simulink model "Progetto_Tesi"  (R2023b)
settings: Solver=VariableStepAuto  StartTime=0.0  StopTime=inf  RelTol=1e-3
StartFcn:
  | model_params
model workspace (MAT data in the model file):
  ax_pre_init = 7
values from neighbouring files (symbols this model uses):
  soglia_nonlin = 0.5    [model_params.m]
undefined symbols (not defined in the file or in its folder): deg, m, s
libraries: qbmove_library x4, CP_library x1, QB_pacer_lib x1
settings Model: Creator=ilari  LastModifiedBy=ilari

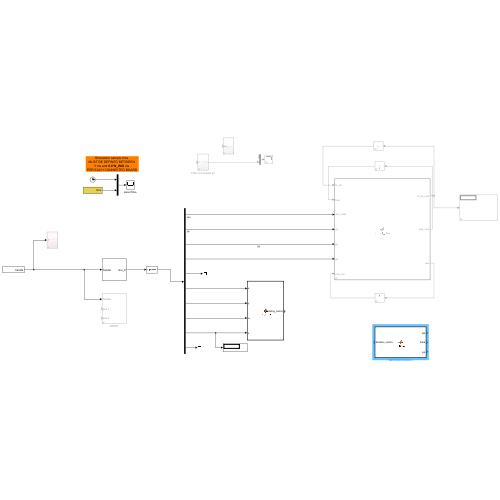
[thumbnail: Simulink's stored preview of the top-level diagram]
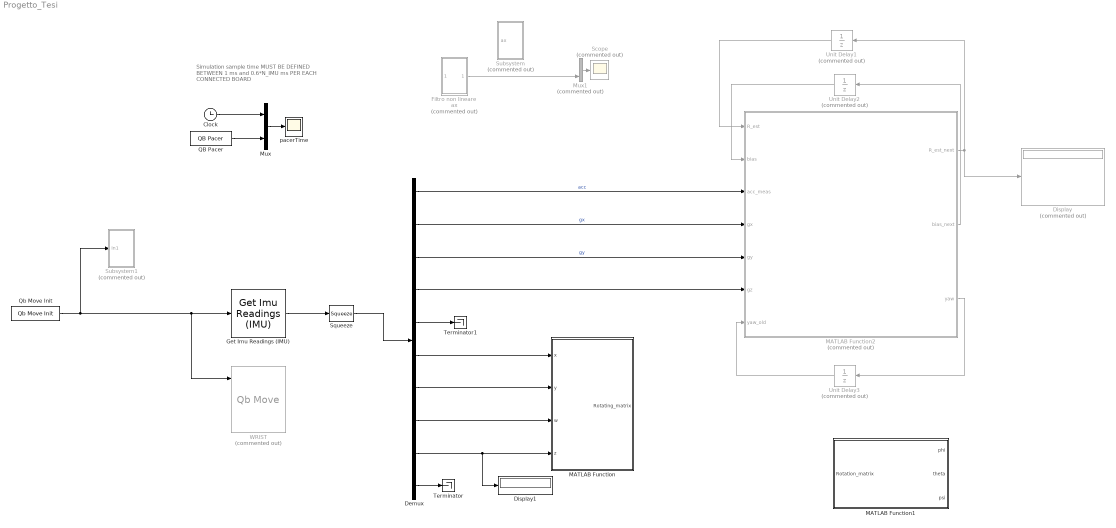
== system Progetto_Tesi ==
  note: Simulation sample time
      | MUST BE DEFINED BETWEEN
      | 1 ms and 0.6*N_IMU ms
      | PER EACH CONNECTED BOARD
  Clock : Clock
  Demux : Demux  Outputs=[3 1 1 1 3 1 1 1 1 1]
  Display : Display  Commented=on
  Display1 : Display
  Filtro non lineare ax : Subsystem  Commented=on
  Get Imu Readings (IMU) : CP_library/Get Imu Readings (IMU)  ID=2  N_IMU=1  DAISY_CHAINING=off  ACC_UNITY=m/(s^2)  GYRO_UNITY=deg/s  MAG_UNITY=uT
      settings: SourceProductName=Centro Piaggio Library
  MATLAB Function : MATLAB Function  TreatAsAtomicUnit=on
  MATLAB Function1 : MATLAB Function  TreatAsAtomicUnit=on
  MATLAB Function2 : MATLAB Function  Commented=on  TreatAsAtomicUnit=on
  Mux : Mux  Inputs=2
  Mux1 : Mux  Commented=on  Inputs=2
  QB Pacer : QB_pacer_lib/QB Pacer  simTimePerRealTime=1
      settings: SourceProductName=QB Pacer
  Qb Move Init : qbmove_library/Qb Move Init  NUMBER_OF_COM='COM9'  BAUD_RATE_COM=2000000
      settings: SourceProductName=Qb Move Library
  Scope : Scope  Commented=on
  Squeeze : Squeeze
  Subsystem : Subsystem  Commented=on
  Subsystem1 : Subsystem  Commented=on
  Terminator : Terminator
  Terminator1 : Terminator
  Unit Delay1 : UnitDelay  Commented=on  SampleTime=-1  HasFrameUpgradeWarning=on
  Unit Delay2 : UnitDelay  Commented=on  SampleTime=-1  HasFrameUpgradeWarning=on
  Unit Delay3 : UnitDelay  Commented=on  SampleTime=-1  HasFrameUpgradeWarning=on
  WRIST : qbmove_library/Qb Move  Commented=on  ID=2  ACTIVE_COMM_DIRECTIONS=Tx  CONTROL_MODE=Prime Movers Positions  DAISY_CHAINING=off  MAX_ANG=0  SW_LIMIT=inf  OFFSET=0  ACTIVATE=on  WDT=0.0  UNIT=TICK
      settings: SourceProductName=Qb Move Library
  pacerTime : Scope
  wires:
  Clock/1 -> Mux/1
  QB Pacer/1 -> Mux/2
  Mux/1 -> pacerTime/1
  Qb Move Init/1 -> Get Imu Readings (IMU)/1, WRIST/1, Subsystem1/1(In1)
  Get Imu Readings (IMU)/1 -> Squeeze/1
  Squeeze/1 -> Demux/1
  Filtro non lineare ax/1(Out1) -> Mux1/2
  Mux1/1 -> Scope/1
  Demux/1 -> MATLAB Function2/3(acc_meas)  "acc"
  Demux/2 -> MATLAB Function2/4(gx)  "gx"
  Demux/3 -> MATLAB Function2/5(gy)  "gy"
  Demux/4 -> MATLAB Function2/6(gz)
  MATLAB Function2/3(yaw) -> Unit Delay3/1
  Unit Delay3/1 -> MATLAB Function2/7(yaw_old)
  MATLAB Function2/2(bias_next) -> Unit Delay2/1
  Unit Delay2/1 -> MATLAB Function2/2(bias)
  Unit Delay1/1 -> MATLAB Function2/1(R_est)
  MATLAB Function2/1(R_est_next) -> Unit Delay1/1, Display/1
  Demux/5 -> Terminator1/1
  Demux/10 -> Terminator/1
  Demux/6 -> MATLAB Function/1(x)
  Demux/7 -> MATLAB Function/2(y)
  Demux/8 -> MATLAB Function/3(w)
  Demux/9 -> Display1/1, MATLAB Function/4(z)

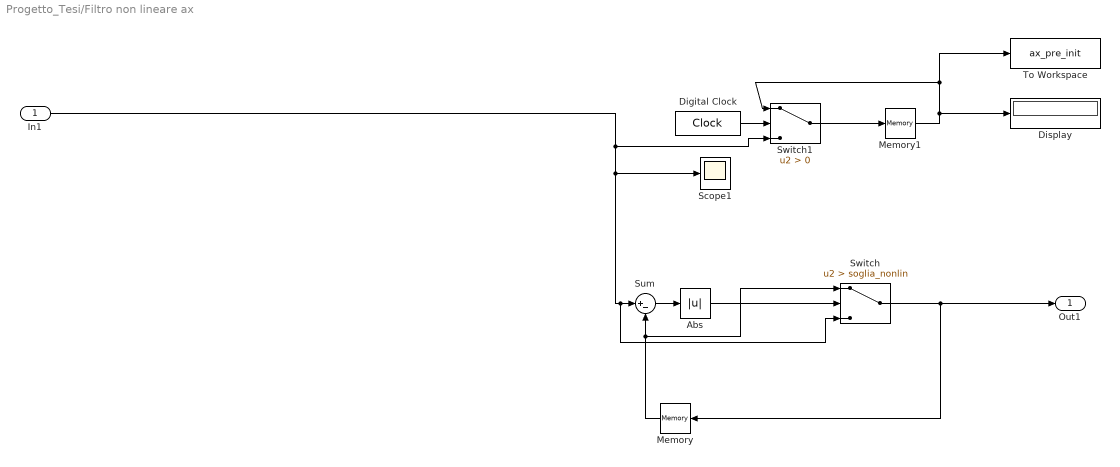
== system Progetto_Tesi/Filtro non lineare ax ==
  In1 : Inport
  Abs : Abs  SaturateOnIntegerOverflow=off
  Digital Clock : DigitalClock
  Display : Display
  Memory : Memory  InitialCondition=ax_pre_init
  Memory1 : Memory
  Scope1 : Scope
  Sum : Sum  Inputs=|+-
  Switch : Switch  Criteria=u2 > Threshold  Threshold=soglia_nonlin  SaturateOnIntegerOverflow=off  InputSameDT=off
  Switch1 : Switch  Criteria=u2 > Threshold  SaturateOnIntegerOverflow=off  InputSameDT=off
  To Workspace : ToWorkspace  VariableName=ax_pre_init  SaveFormat=Timeseries  SampleTime=-1
  Out1 : Outport
  wires:
  Switch/1 -> Out1/1, Memory/1
  Memory/1 -> Sum/2, Switch/1
  In1/1 -> Switch1/3, Switch/3, Sum/1, Scope1/1
  Abs/1 -> Switch/2
  Sum/1 -> Abs/1
  Switch1/1 -> Memory1/1
  Memory1/1 -> Switch1/1, To Workspace/1, Display/1
  Digital Clock/1 -> Switch1/2

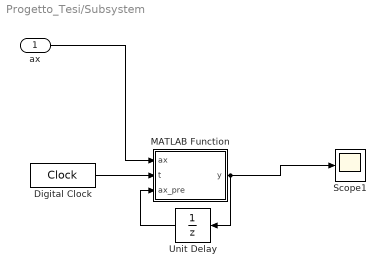
== system Progetto_Tesi/Subsystem ==
  ax : Inport
  Digital Clock : DigitalClock
  MATLAB Function : MATLAB Function  TreatAsAtomicUnit=on
  Scope1 : Scope
  Unit Delay : UnitDelay  SampleTime=-1  HasFrameUpgradeWarning=on
  wires:
  MATLAB Function/1(y) -> Unit Delay/1, Scope1/1
  Digital Clock/1 -> MATLAB Function/2(t)
  Unit Delay/1 -> MATLAB Function/3(ax_pre)
  ax/1 -> MATLAB Function/1(ax)

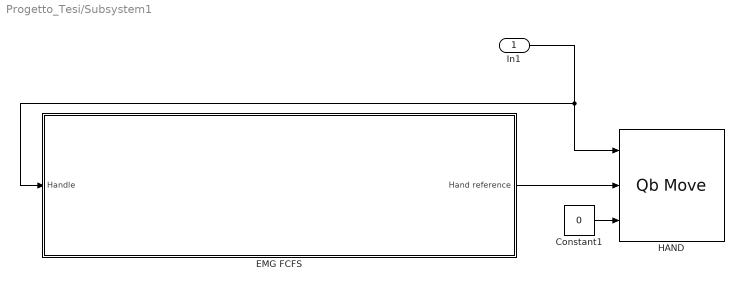
== system Progetto_Tesi/Subsystem1 ==
  In1 : Inport
  Constant1 : Constant  Value=0
  EMG FCFS : Subsystem
  HAND : qbmove_library/Qb Move  ID=1  ACTIVE_COMM_DIRECTIONS=Tx  CONTROL_MODE=Prime Movers Positions  DAISY_CHAINING=off  MAX_ANG=0  SW_LIMIT=inf  OFFSET=0  ACTIVATE=on  WDT=0.0  UNIT=TICK
      settings: SourceProductName=Qb Move Library
  wires:
  In1/1 -> HAND/1, EMG FCFS/1(Handle)
  Constant1/1 -> HAND/3
  EMG FCFS/1(Hand reference) -> HAND/2

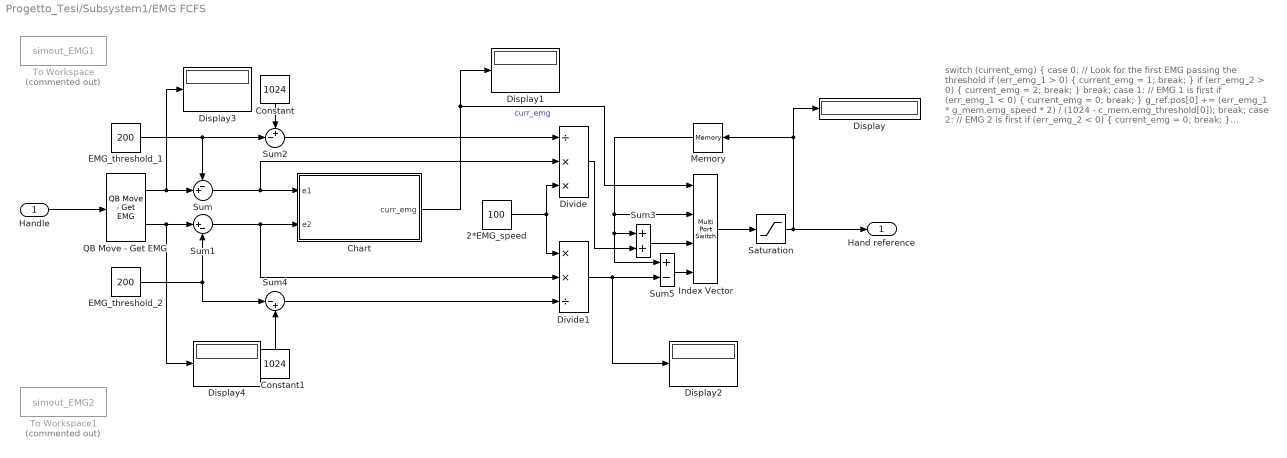
== system Progetto_Tesi/Subsystem1/EMG FCFS ==
  note: switch (current_emg) {
      | case 0:
      | // Look for the first EMG passing the threshold
      | if (err_emg_1 > 0) {
      | current_emg = 1;
      | break;
      | }
      | if (err_emg_2 > 0) {
      | current_emg = 2;
      | break;
      | }
      | break;
      |
      | case 1:
      | // EMG 1 is first
      | if (err_emg_1 < 0) {
      | current_emg = 0;
      | break;
      | }
      | g_ref.pos[0] += (err_emg_1 * g_mem.emg_speed * 2) / (1024 - c_mem.emg_threshold[0]);
      | break;
      |
      | case 2:
      | // EMG 2 is first
      | if (err_emg_2 < 0) {
      | current_emg = 0;
      | break;
      | }
      | g_ref.pos[0] -= (err_emg_2 * g_mem.emg_speed * 2) / (1024 - c_mem.emg_threshold[1]);
      | break;
      |
      | default:
      | break;
      | }
  Handle : Inport
  2*EMG_speed : Constant  Value=100
  Chart : Stateflow chart  TreatAsAtomicUnit=on
  Constant : Constant  Value=1024
  Constant1 : Constant  Value=1024
  Display{,1..4} (5 alike) : Display
      Display settings: Format=decimal (Stored Integer)
  Divide : Product  Inputs=/**
  Divide1 : Product  Inputs=**/
  EMG_threshold_1 : Constant  Value=200
  EMG_threshold_2 : Constant  Value=200
  Index Vector : MultiPortSwitch  DataPortOrder=Zero-based contiguous  zeroidx=on  SaturateOnIntegerOverflow=off  InputSameDT=off
  Memory : Memory
  QB Move - Get EMG : qbmove_library/QB Move - Get EMG  ID=2  DAISY_CHAINING=off
      settings: SourceProductName=Qb Move Library
  Saturation : Saturate  UpperLimit=19000  LowerLimit=0
  Sum : Sum  Inputs=-+|
  Sum1 : Sum  Inputs=|+-
  Sum2 : Sum  Inputs=+-|
  Sum3 : Sum
  Sum4 : Sum  Inputs=|-+
  Sum5 : Sum  Inputs=+-
  To Workspace : ToWorkspace  Commented=on  VariableName=simout_EMG1  SaveFormat=Timeseries  SampleTime=-1
  To Workspace1 : ToWorkspace  Commented=on  VariableName=simout_EMG2  SaveFormat=Timeseries  SampleTime=-1
  Hand reference : Outport
  wires:
  Memory/1 -> Index Vector/2, Sum5/1, Sum3/1
  Sum5/1 -> Index Vector/4
  Sum1/1 -> Divide1/2, Chart/2(e2)
  2*EMG_speed/1 -> Divide1/1, Divide/3
  Constant1/1 -> Sum4/2
  Chart/1(curr_emg) -> Display1/1, Index Vector/1  "curr_emg"
  Sum3/1 -> Index Vector/3
  Sum/1 -> Divide/2, Chart/1(e1)
  Index Vector/1 -> Saturation/1
  QB Move - Get EMG/1 -> Display3/1, Sum/2
  Sum4/1 -> Divide1/3
  Divide/1 -> Sum3/2
  Constant/1 -> Sum2/1
  EMG_threshold_1/1 -> Sum2/2, Sum/1
  Divide1/1 -> Display2/1, Sum5/2
  Handle/1 -> QB Move - Get EMG/1
  QB Move - Get EMG/2 -> Display4/1, Sum1/1
  Sum2/1 -> Divide/1
  Saturation/1 -> Hand reference/1, Display/1, Memory/1
  EMG_threshold_2/1 -> Sum4/1, Sum1/2

== matlab function Progetto_Tesi/MATLAB Function ==
  data: x input; Rotating_matrix output; y input; w input; z input
function Rotating_matrix = Quat2rot(x , y , w ,z)

Rotating_matrix = [(1 - 2*(y^2 + z^2)) , 2*(x*y - w*z) , 2*(w*y + x*z);
                    2*(x*y + w*z) , (1 - 2*(x^2 + z^2)) , 2*(y*z - w*x);
                    2*(x*z - w*y) , 2*(w*x + y*z) , (1 - 2*(x^2 + y^2))];
end

== matlab function Progetto_Tesi/Subsystem/MATLAB Function ==
  data: ax input; y output; t input; ax_pre input
function y = fcn(ax , t, ax_pre)

if t < 1
    ax_pre = ax;
end


if abs(ax-ax_pre)> 2
    y = ax_pre;
else 
    y = ax;

end

ax_pre = ax;

== stateflow chart Progetto_Tesi/Subsystem1/EMG FCFS/Chart ==
  state State0
    entry: curr_emg = 0;
  state State1
    entry: curr_emg = 1;
  state State2
    entry: curr_emg = 2;
  (default) -> State0
  State0 -> State1 [order 1] : [e1 > 0]
  State1 -> State0 : [e1 < 0]
  State2 -> State0 : [e2 < 0]
  State0 -> State2 [order 2] : [e2 > 0]
  data: e1 input; e2 input; curr_emg output

== matlab function Progetto_Tesi/MATLAB Function2 ==
  data: R_est input; R_est_next output; bias input; acc_meas input; gx input; gy input; gz input; yaw_old input; bias_next output; yaw output
function [ R_est_next, bias_next, yaw] = explicit_filter(  R_est , bias , acc_meas, gx, gy, gz, yaw_old)  

    omega_meas = [gx ; gy ; gz];
    
    k_corr = 0.5; 
    K_bias = diag([0.1 0.1 0.36]);
    K_acc = 1; %[s^4 / rad^2]
    sample_time = 0.01; % poi c'è da mettere la cosa dei parametri
   
    inertial_dir = [0; 0; 9.81]; %[3 x 1]
    acc_est = R_est' * inertial_dir; %[3 x 1]

    % Explicit filter implementation in discrete time with Rodrigue's
    % formula to compute A_k matrix
    % Discrete Formulation: R_est(k+1) = R_est(k)*A_k
    
    % Normalize estimated and measured acceleration to compute correction
    % term
    acc_est  = acc_est/norm(acc_est); %[3 x 1]
    acc_meas = acc_meas/norm(acc_meas); %[3 x 1]

    % Correction term
    w_corr = K_acc * cross(acc_meas, acc_est);
    
    % Bias estimation
    
   
    bias_next =  bias - sample_time * K_bias * w_corr;  
    

    disp(class(bias_next));
    % Estimate next orientation matrix
    A = omega_meas - bias + k_corr*w_corr;
	R_est_next = R_est * rodrigue_formula(A, sample_time);

   %eul = dcm2angle(R_est', 'ZYX');
    
     % eul = rotm2eul(R_est);
     % roll = rad2deg(eul(1));
     % pitch = rad2deg(eul(2));
     yaw = rad2deg(yaw_old + sample_time*(omega_meas(3) - bias(2)));
     ciao = sample_time*(omega_meas(3) - bias(2));
     disp(ciao);
end

function Y = rodrigue_formula( omega, T )
    % Given as input a vector of three elements, omega, and a time period
    % T, this function computes the exponential matrix exp( skew(omega), T
    % ), using the Rodrigue's formula. skew() is the skew symmetric
    % operator.

    term1 = eye(3);
	term2 = skew( omega )*sin( norm(omega)*T )/norm(omega);
	term3 = ( skew( omega )^2 )*( 1 - cos( norm(omega)*T ) )/( norm(omega)^2 );
	Y = term1 + term2 + term3;
end

function Y = skew( u )
  % Given in input a vector of three elements, this function computes the
  % relative 3x3 skew symmetric matrix.
  %      |x|    | 0 -z  y |
  % skew(|y|) = | z  0 -x |
  %      |z|    |-y  x  0 |

    Y = zeros(3);
    Y = [0 -u(3) u(2); u(3) 0 -u(1); -u(2) u(1) 0];
end

== matlab function Progetto_Tesi/MATLAB Function1 ==
  data: Rotation_matrix input; phi output; theta output; psi output
function [phi , theta , psi] = Rot2eul(Rotation_matrix)


% Verifico che la matrice R sia 3x3

assert(all(size(R) == [3 3]), 'La matrice di rotazione deve essere 3x3');

% Calcolo dell'angolo theta

R31 = R(3,1);

if R31 ~= 1 && R31 ~= -1
    theta1 = -asin(R31);
    theta2 = pi - theta1;
end

%%

cos_theta1 = cos(theta1);
cos_theta2 = cos(theta2);
    
if cos(theta1) ~= 0
    psi1 = atan2(R(3,2) / cos_theta1, R(3,3) / cos_theta1);
    phi1 = atan2(R(2,1) / cos_theta1, R(1,1) / cos_theta1);

else
    % Caso speciale di gimbal lock
    psi1 = atan2(R(1,2), R(1,3));
    phi1 = 0;
end

if abs(cos_theta2) > eps
    psi2 = atan2(R(3,2) / cos_theta2, R(3,3) / cos_theta2);
    phi2 = atan2(R(2,1) / cos_theta2, R(1,1) / cos_theta2);
else
    % Caso speciale di gimbal lock
    psi2 = atan2(R(1,2), R(1,3));
    phi2 = 0;
end

%%

% Seleziona una soluzione. Qui puoi scegliere di restituire entrambe o solo una
psi = psi1;  % o psi2
theta = theta1;  % o theta2
phi = phi1;  % o phi2
